simulink model "Adaptive_Impedance"  (R2023b)
settings: Solver=VariableStepAuto  StartTime=0.0  StopTime=10.0  RelTol=1e-3
settings Model: Creator=91996  LastModifiedBy=91996

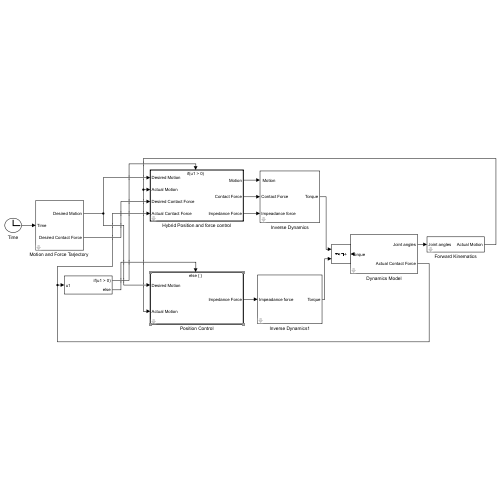
[thumbnail: Simulink's stored preview of the top-level diagram]
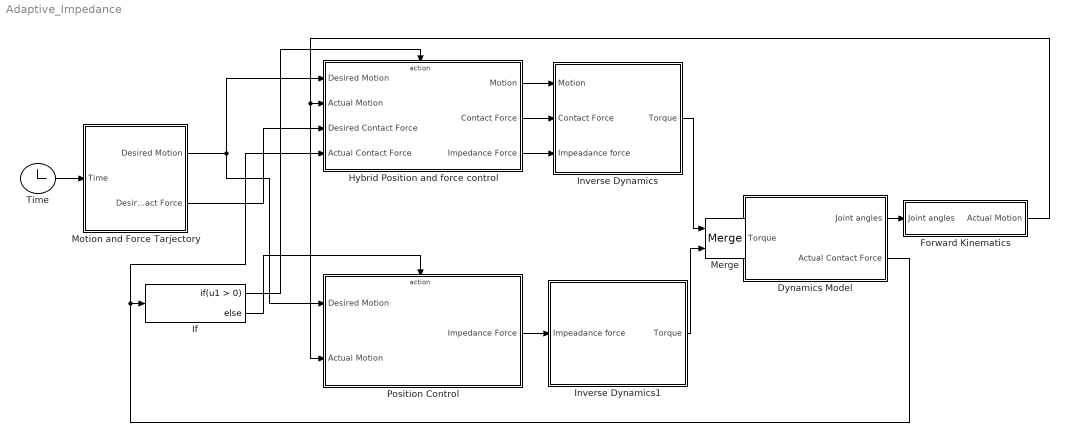
== system Adaptive_Impedance ==
  Dynamics Model : Subsystem
      mask DialogControl C Prompt: Parameters
  Forward Kinematics : Subsystem
      mask DialogControl Kinematics Prompt: Parameters
  Hybrid Position and force control : Subsystem
      mask DialogControl A Prompt: Parameters
  If : If
  Inverse Dynamics : Subsystem
      mask DialogControl B Prompt: Parameters
  Inverse Dynamics1 : Subsystem
      mask DialogControl B Prompt: Parameters
  Merge : Merge
  "Motion and Force Tarjectory " : Subsystem
      mask DialogControl E Prompt: Parameters
  Position Control : Subsystem
      mask DialogControl A Prompt: Parameters
  Time : Clock
  wires:
  "Motion and Force Tarjectory "/1(Desired Motion) -> Hybrid Position and force control/1(Desired Motion), Position Control/1(Desired Motion)
  Hybrid Position and force control/1(" Motion") -> Inverse Dynamics/1(" Motion")
  Time/1 -> "Motion and Force Tarjectory "/1(Time)
  Forward Kinematics/1(Actual Motion) -> Position Control/2(Actual Motion), Hybrid Position and force control/2(Actual Motion)
  Dynamics Model/1(Joint angles) -> Forward Kinematics/1(Joint angles)
  "Motion and Force Tarjectory "/2(Desired Contact Force) -> Hybrid Position and force control/3(Desired Contact Force)
  Hybrid Position and force control/2(Contact Force) -> Inverse Dynamics/2(Contact Force)
  Hybrid Position and force control/3(Impedance Force) -> Inverse Dynamics/3(Impeadance force)
  Dynamics Model/2(Actual Contact Force) -> Hybrid Position and force control/4(Actual Contact Force), If/1
  If/1 -> Hybrid Position and force control/Action
  If/2 -> Position Control/Action
  Position Control/1(Impedance Force) -> Inverse Dynamics1/1(Impeadance force)
  Merge/1 -> Dynamics Model/1(Torque)
  Inverse Dynamics1/1(Torque) -> Merge/2
  Inverse Dynamics/1(Torque) -> Merge/1

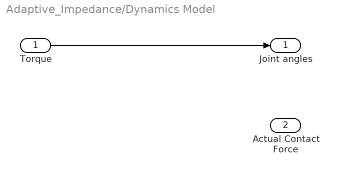
== system Adaptive_Impedance/Dynamics Model ==
  Torque : Inport
  Joint angles : Outport
  Actual Contact Force : Outport  Port=2
  wires:
  Torque/1 -> Joint angles/1

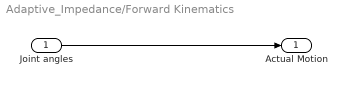
== system Adaptive_Impedance/Forward Kinematics ==
  Joint angles : Inport
  Actual Motion : Outport
  wires:
  Joint angles/1 -> Actual Motion/1

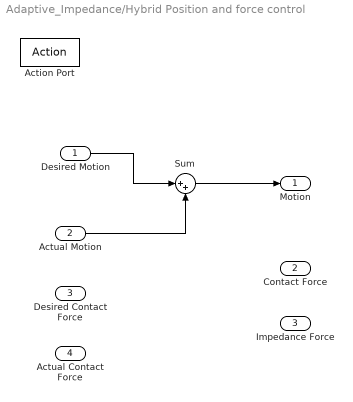
== system Adaptive_Impedance/Hybrid Position and force control ==
  Desired Motion : Inport
  Actual Motion : Inport  Port=2
  Desired Contact Force : Inport  Port=3
  Actual Contact Force : Inport  Port=4
  Action Port : ActionPort  ActionPortLabel=if(u1 > 0)
  Sum : Sum  Inputs=|++
  " Motion" : Outport
  Contact Force : Outport  Port=2
  Impedance Force : Outport  Port=3
  wires:
  Desired Motion/1 -> Sum/1
  Actual Motion/1 -> Sum/2
  Sum/1 -> " Motion"/1

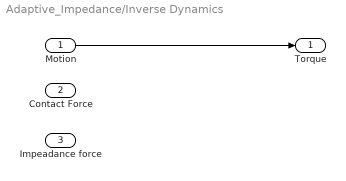
== system Adaptive_Impedance/Inverse Dynamics ==
  " Motion" : Inport
  Contact Force : Inport  Port=2
  Impeadance force : Inport  Port=3
  Torque : Outport
  wires:
  " Motion"/1 -> Torque/1

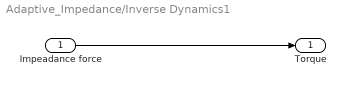
== system Adaptive_Impedance/Inverse Dynamics1 ==
  Impeadance force : Inport
  Torque : Outport
  wires:
  Impeadance force/1 -> Torque/1

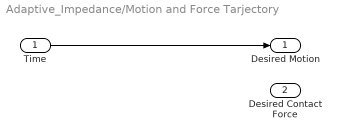
== system Adaptive_Impedance/Motion and Force Tarjectory  ==
  Time : Inport
  Desired Motion : Outport
  Desired Contact Force : Outport  Port=2
  wires:
  Time/1 -> Desired Motion/1

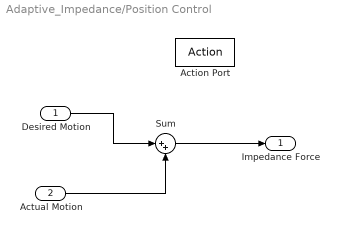
== system Adaptive_Impedance/Position Control ==
  Desired Motion : Inport
  Actual Motion : Inport  Port=2
  Action Port : ActionPort  ActionPortLabel=else
  Sum : Sum  Inputs=|++
  Impedance Force : Outport
  wires:
  Desired Motion/1 -> Sum/1
  Actual Motion/1 -> Sum/2
  Sum/1 -> Impedance Force/1
